simulink model "Robot_Simulink_Continous"  (R2018b)
settings: Solver=FixedStepAuto  StartTime=0.0  StopTime=Tt  FixedStep=Ts  RelTol=1e-3
values from neighbouring files (symbols this model uses):
  b = 0.25    [KF.m]    (also in Robot.m = 0.5)
  R_wl = 0.5    [KF.m]    (also in Robot.m = 0.35)
  R_wr = 0.5    [KF.m]    (also in Robot.m = 0.35)
  theta0 = pi/2    (= 1.57079632679)    [KF.m]    (also in Robot.m = 0.785398163397)
  u_wl = pi/2    (= 1.57079632679)    [KF.m]    (also in Robot.m)
  u_wr = pi/4    (= 0.785398163397)    [KF.m]    (also in Robot.m = 1.57079632679)
  x0 = 0    [KF.m]    (also in Robot.m)
  y0 = 0    [KF.m]    (also in Robot.m)
settings Model: Creator=Sergio  LastModifiedBy=Sergio

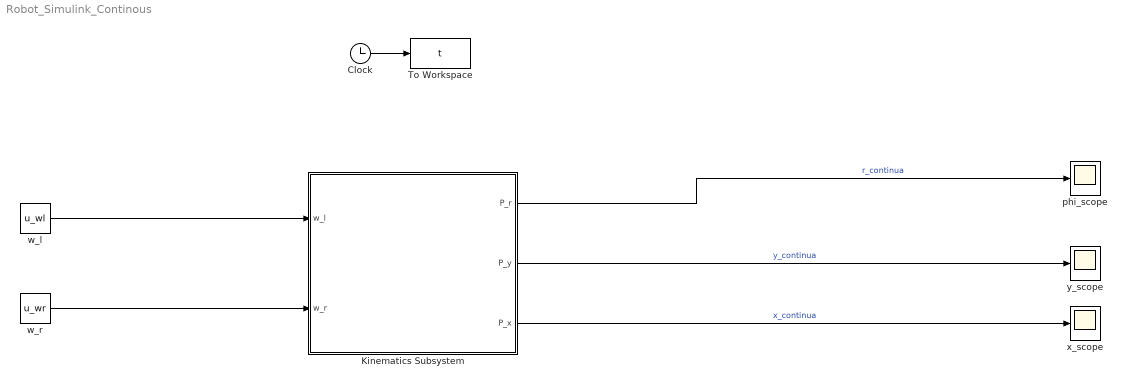
== system Robot_Simulink_Continous ==
  Clock : Clock
  Kinematics Subsystem : Subsystem
      mask Display: image('D:\Máster Robótica y Automatización - msi\Asignaturas\Segundo cuatrimestre\Asignaturas\2.- Robots Móviles\2_ Material docente\Practicas\2018 -2019\Pr1 - Kalman Filter\Imagenes\Passive-Stability1.png');
  To Workspace : ToWorkspace  VariableName=t  SampleTime=-1
  phi_scope : Scope
  "w_l " : Constant  Value=u_wl
  "w_r " : Constant  Value=u_wr
  "x_scope " : Scope
  "y_scope " : Scope
  wires:
  "w_r "/1 -> Kinematics Subsystem/2(w_r)
  "w_l "/1 -> Kinematics Subsystem/1("w_l ")
  Clock/1 -> To Workspace/1
  Kinematics Subsystem/1(P_r) -> phi_scope/1  "r_continua"
  Kinematics Subsystem/2(P_y) -> "y_scope "/1  "y_continua"
  Kinematics Subsystem/3(P_x) -> "x_scope "/1  "x_continua"

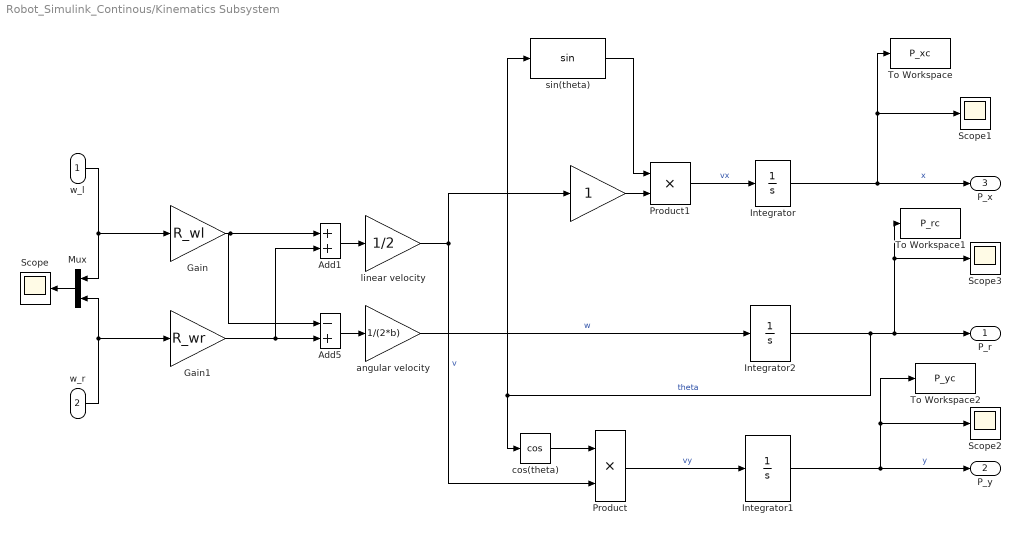
== system Robot_Simulink_Continous/Kinematics Subsystem ==
  "w_l " : Inport
  w_r : Inport  Port=2
  " " : Gain
  Add1 : Sum
  Add5 : Sum  Inputs=-+
  Gain : Gain  Gain=R_wl
  Gain1 : Gain  Gain=R_wr
  Integrator : Integrator  InitialCondition=x0
  Integrator1 : Integrator  InitialCondition=y0
  Integrator2 : Integrator  InitialCondition=theta0
  Mux : Mux  Inputs=2
  Product : Product
  Product1 : Product
  Scope{,1..3} (4 alike) : Scope
  To Workspace : ToWorkspace  VariableName=P_xc  SampleTime=-1
  To Workspace1 : ToWorkspace  VariableName=P_rc  SampleTime=-1
  To Workspace2 : ToWorkspace  VariableName=P_yc  SampleTime=-1
  angular velocity : Gain  Gain=1/(2*b)
  cos(theta) : Trigonometry  Operator=cos
  linear velocity : Gain  Gain=1/2
  sin(theta) : Trigonometry
  P_r : Outport
  P_y : Outport  Port=2
  P_x : Outport  Port=3
  wires:
  " "/1 -> Product1/2
  Mux/1 -> Scope/1
  Product/1 -> Integrator1/1  "vy"
  Product1/1 -> Integrator/1  "vx"
  w_r/1 -> Gain1/1, Mux/2
  "w_l "/1 -> Mux/1, Gain/1
  linear velocity/1 -> Product/2, " "/1  "v"
  sin(theta)/1 -> Product1/1
  Integrator2/1 -> P_r/1, To Workspace1/1, Scope3/1, sin(theta)/1, cos(theta)/1  "theta"
  angular velocity/1 -> Integrator2/1  "w"
  Integrator1/1 -> P_y/1, Scope2/1, To Workspace2/1  "y"
  Integrator/1 -> P_x/1, To Workspace/1, Scope1/1  "x"
  Add1/1 -> linear velocity/1
  Gain/1 -> Add5/1, Add1/1
  Gain1/1 -> Add1/2, Add5/2
  Add5/1 -> angular velocity/1
  cos(theta)/1 -> Product/1
